simulink model "PLL_type2"  (R2014b)
settings: Solver=VariableStepDiscrete  StartTime=0.0  StopTime=50000/fs  RelTol=1e-3
PreLoadFcn:
  | %%%%%%%%%%%%%%%%%%%%%%%%%%%%%%%%%%%%%%%%%%%%%%%%%%%%%%%%%%%%%%%%%%%%%%%%%%%
  | % check to see if Simulink library folder is missing from the MATLAB path %
  | %%%%%%%%%%%%%%%%%%%%%%%%%%%%%%%%%%%%%%%%%%%%%%%%%%%%%%%%%%%%%%%%%%%%%%%%%%%
  | if isempty(strfind(path, 'rtlsdr_book_library'))
  | 
  |     % create error window
  |     fig_error = figure(...
  |         'Name', 'Error: RTL-SDR Book Library',...
  |         'Toolbar','none',...
  |         'MenuBar','none',...
  |         'NumberTitle','off',...
  |         'Resize','off',...
  |         'WindowStyle','modal');
  |     fig_error.Position(3) = 600;
  |     fig_error.Position(4) = 150;
  |     fig_axes = axes(...
  |         'Parent',fig_error,...
  |         'Position',[0,0,1,1],...
  |         'visible','off');
  |     % error message
  |     t_title = text(.05,.8,...
  |         'MISSING DIRECTORIES',...
  |         'FontSize',11.5);
  |     t_body = text(.075,.6,...
  |         [{'Simulink cannot find the  \it{<root>}\rm / \it{rtlsdr\_book\_library}\rm  folder in the \it{MATLAB Path}\rm.'},...
  |         {'Please set the MATLAB path following the instructions given in Exercise 2.4.'}],...
  |         'FontSize',10.5);
  |     % buttons
  |     btn_path = uicontrol(...
  |         'Parent',fig_error,...
  |         'String','Set Path Now',...
  |         'FontSize',10,...
  |         'Callback', 'pathtool; close(fig_error);',...
  |         'Position', [fig_error.Position(3)/2-210, 30, 200, 30]);
  |     btn_abort = uicontrol(...
  |         'Parent',fig_error,...
  |         'String','No thanks',...
  |         'FontSize',10,...
  |         'Callback', 'close(fig_error); abort=1;',...
  |         'Position', [fig_error.Position(3)/2+10, 30, 200, 30]);
  | 
  |     % pause to allow user to interact with error box
  |     uiwait(fig_error);
  | 
  |     % abort simulation
  |     try
  |         if abort==1
  |             set_param(gcs, 'SimulationCommand', 'stop');
  |         end
  |     end
  | 
  |     % if user has set path, allow diagram to be updated
  |     if ~exist('abort','var')
  |         % create error window
  |         fig_update = figure(...
  |             'Name', 'Update Diagram',...
  |             'Toolbar','none',...
  |             'MenuBar','none',...
  |             'NumberTitle','off',...
  |             'Resize','off');
  |         fig_update.Position(3) = 400;
  |         fig_update.Position(4) = 120;
  |         fig_axes = axes(...
  |             'Parent',fig_update,...
  |             'Position',[0,0,1,1],...
  |             'visible','off');
  |         % instruction message
  |         t_body = text(.075,.7,...
  |             'Once you have set the path, update the block diagram',...
  |             'FontSize',10.5);
  |         % button
  |         btn_update = uicontrol(...
  |             'Parent',fig_update,...
  |             'String','Update Block Diagram',...
  |             'FontSize',10,...
  |             'Callback', 'set_param(gcs,''SimulationCommand'',''update''); close(gcf)',...
  |             'Position', [fig_update.Position(3)/2-100, 30, 200, 30]);
  |     end
  | 
  |     % clear error components
  |     clear('fig_error','fig_update','fig_axes','t_title','t_body','btn_path','btn_abort','btn_update','abort');
  | 
  | end
  | %%%%%%%%%%%%%%%%%%%%%%%%%%%%%%%%%%%%%%%%%%%%%%%%%%%%%%%%%%%%%%%%%%%%%%%%%%%
  | 
  | 
  | MHz = 100;
  | fs = MHz * 1e6;
StartFcn:
  | close all;
StopFcn:
  | doFFTplot(fs, [Synthesised(round(length(Synthesised)*0.9):end), Error(round(length(Error)*0.9):end), Reference(round(length(Reference)*0.9):end)], ['Synthesised'; 'Error      '; 'Reference  '], 1, 7, 'hann');
  | set(7,'Name','FFT Plots of Input and Synthesised Sine Waves (Final 10% of Simulation Time)','NumberTitle','off');
  | setStandardFigSize(7);
  | legend('Error','Synthesised','Reference','location','NorthEast');
  | 
  | figure(8)
  | plot(1e6*Inst_freq.time,1e-6*Inst_freq.signals.values,'m');
  | xlabel('Time (\mus)');
  | ylabel('Frequency (MHz)');
  | title('PLL Adapting');
  | grid on;
  | 
  | set(8,'Name','Frequency Generated by VCO','NumberTitle','off');
  | setStandardFigSize(8);
undefined symbols (not defined in the file): startfcn_time_scope
libraries: commsynccomp2 x2, simulink x1, rtlsdr_book_library x1
CloseFcn:
  | closefcn_model;
Description:
  | Software, Simulation Examples and Design Exercises Licence Agreement
  | 
  | This license agreement refers to the simulation examples, design exercises and files,
  | and associated software MATLAB and Simulink resources that accompany the book:
  | 
  |      Title: Software Defined Radio using MATLAB & Simulink and the RTL-SDR
  |      Published by Strathclyde Academic Media, 2015
  |      Authored by Robert W. Stewart, Kenneth W. Barlee, Dale S.W. Atkinson,
  |      and Louise H. Crockett
  | 
  | and made available as a download from, www.desktopSDR.com or variously acquired
  | by other means such as via USB storage, cloud storage, disk or any other electronic
  | or optical or magnetic storage mechanism. These files and associated software may
  | be used subject to the terms of agreement of the conditions below:
  | 
  |     Copyright © 2015 Robert W. Stewart, Kenneth W. Barlee, Dale S.W. Atkinson,
  |     and Louise H. Crockett
  |     All rights reserved.
  | 
  | Redistribution and use in source and binary forms, with or without modification, are
  | permitted provided that the following conditions are met:
  | 
  |    1.  Redistributions of source code must retain the above copyright notice, this list of
  |         conditions and the following disclaimer.
  | 
  |    2.  Redistributions in binary form must reproduce the above copyright notice, this
  |         list of conditions and the following disclaimer in the documentation and/or other
  |         materials provided with the distribution.
  | 
  |    3.  Neither the name of the copyright holder nor the names of its contributors may
  |         be used to endorse or promote products derived from this software without
  |         specific prior written permission.
  | 
  |    4.  In all cases, the software is, and all modifications and derivatives of the
  |         software shall be, licensed to you solely for use in conjunction with The
  |         MathWorks, Inc. products and service offerings.
  | 
  | THIS SOFTWARE IS PROVIDED BY THE COPYRIGHT HOLDERS AND CONTRIBUTORS
  | "AS IS" AND ANY EXPRESS OR IMPLIED WARRANTIES, INCLUDING, BUT NOT LIMITED
  | TO, THE IMPLIED WARRANTIES OF MERCHANTABILITY AND FITNESS FOR A
  | PARTICULAR PURPOSE ARE DISCLAIMED. IN NO EVENT SHALL THE COPYRIGHT
  | HOLDER OR CONTRIBUTORS BE LIABLE FOR ANY DIRECT, INDIRECT, INCIDENTAL,
  | SPECIAL, EXEMPLARY, OR CONSEQUENTIAL DAMAGES (INCLUDING, BUT NOT
  | LIMITED TO, PROCUREMENT OF SUBSTITUTE GOODS OR SERVICES; LOSS OF USE,
  | DATA, OR PROFITS; OR BUSINESS INTERRUPTION) HOWEVER CAUSED AND ON ANY
  | THEORY OF LIABILITY, WHETHER IN CONTRACT, STRICT LIABILITY, OR TORT
  | (INCLUDING NEGLIGENCE OR OTHERWISE) ARISING IN ANY WAY OUT OF THE USE
  | OF THIS SOFTWARE, EVEN IF ADVISED OF THE POSSIBILITY OF SUCH DAMAGE.
  | 
  | 
  | Audio Tracks used in Simulations Examples and Design Exercises
  | 
  | The music and vocal files used within the Examples files and software within the book
  | were variously written, arranged, performed, recorded and produced by Garrey Rice,
  | Adam Struth, Jamie Struth, Iain Thistlethwaite and also Marshall Craigmyle who
  | collectively, and individually where appropriate, assert and retain all of their copyright,
  | performance and artistic rights. Permission to use and reproduce this music is
  | granted for all purposes associated with MATLAB and Simulink software and the
  | simulation examples and design exercises files that accompany this book. Requests to
  | use the music for any other purpose should be directed to: info@desktopSDR.com.
  | For information on music track names, full credits, and links to the musicians please
  | refer to www.desktopSDR.com/more/audio.
settings Model: Creator=desktopSDR Team  LastModifiedBy=desktopSDR Team
settings DataIOCC: LimitDataPoints=off  SaveOutput=off  SignalLogging=off  SaveTime=off
settings DebuggingCC: UnderspecifiedInitializationDetection=Classic  MergeDetectMultiDrivingBlocksExec=none

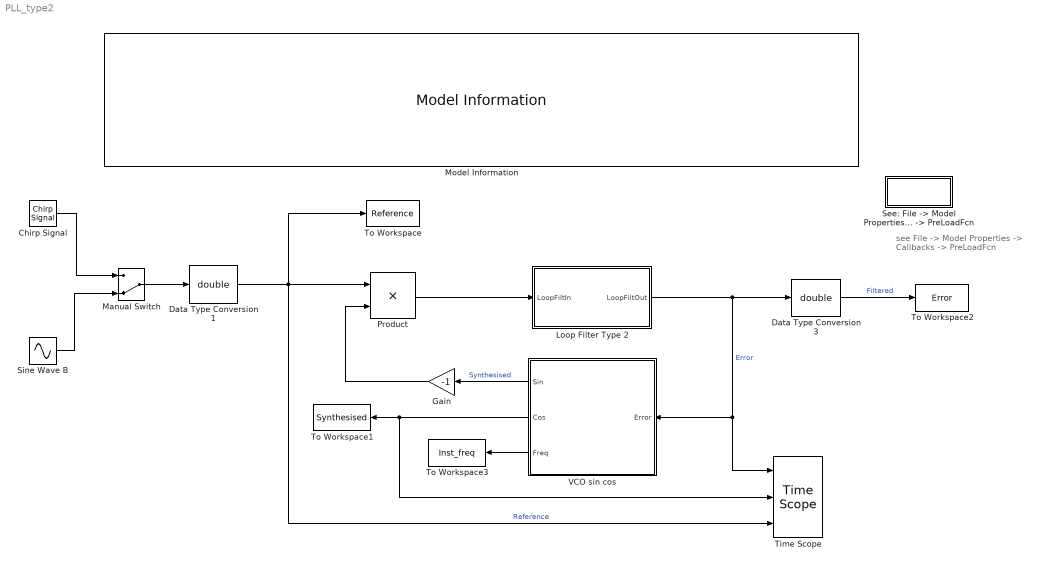
== system PLL_type2 ==
  note: see File -> Model Properties
      | -> Callbacks -> PreLoadFcn
  Chirp Signal : simulink/Sources/Chirp Signal  f1=3.6e6  T=100e3/fs  f2=3.8e6
  Data Type Conversion1 : DataTypeConversion  OutDataTypeStr=double  SampleTime=1/fs
  Data Type Conversion3 : DataTypeConversion  OutDataTypeStr=double  SampleTime=1/fs
  Gain : Gain  Gain=-1
  Loop Filter Type 2 : Subsystem  mask(Loop Filter (Type 2)){K1=0.03125, K2=1.25e-4}
      mask prompts: K1 "K1 (proportional path)"; K2 "K2 (integral path)"
      mask help: This loop filter contains two paths: a proportional path with scaling coefficient K1, and an integral path with scaling coefficient K2.
  Manual Switch : ManualSwitch  CurrentSetting=0
  Model Information : rtlsdr_book_library/Additional Tools/Model Information/Model Information
  Product : Product
  "See: File -> Model Properties -> Callbacks -> PreLoadFcn " : Subsystem
      mask Display:
      | MHz = evalin('base', 'MHz');
      | fprintf(['fs = ',num2str(MHz),' MHz']);
  Sine Wave B : Sin  Frequency=2*pi*3.55e6  Phase=pi/5  SampleTime=0
  Time Scope : TimeScope  StartFcn=startfcn_time_scope;  DefaultConfigurationName=spbscopes.TimeScopeBlockCfg  NumInputPorts=3
  To Workspace : ToWorkspace  VariableName=Reference  SampleTime=-1
  To Workspace1 : ToWorkspace  VariableName=Synthesised  SampleTime=-1
  To Workspace2 : ToWorkspace  VariableName=Error  SampleTime=-1
  To Workspace3 : ToWorkspace  VariableName=Inst_freq  SaveFormat=Structure With Time  SampleTime=-1
  VCO sin cos : Subsystem  mask(Quadratude VCO){fq=3.5e6, sensitivity=1e6}
      mask prompts: fq "Quiescent Frequency (Hz)"; sensitivity "Sensitivity (Hz/V)"
      mask help: This VCO provides both cosine and sine outputs. The quiescent frequency and sensitivity of the VCO can be defined via the mask (and these apply to both sine and cosine outputs). The block also provides the instantaneous frequency as an output.
  wires:
  Data Type Conversion1/1 -> Time Scope/3, Product/1, To Workspace/1  "Reference"
  Data Type Conversion3/1 -> To Workspace2/1  "Filtered"
  Loop Filter Type 2/1(LoopFiltOut) -> VCO sin cos/1(Error), Time Scope/1, Data Type Conversion3/1  "Error"
  Sine Wave B/1 -> Manual Switch/2
  Manual Switch/1 -> Data Type Conversion1/1
  Chirp Signal/1 -> Manual Switch/1
  Product/1 -> Loop Filter Type 2/1(LoopFiltIn)
  VCO sin cos/3(Freq) -> To Workspace3/1
  VCO sin cos/2(Cos) -> Time Scope/2, To Workspace1/1
  VCO sin cos/1(Sin) -> Gain/1  "Synthesised"
  Gain/1 -> Product/2

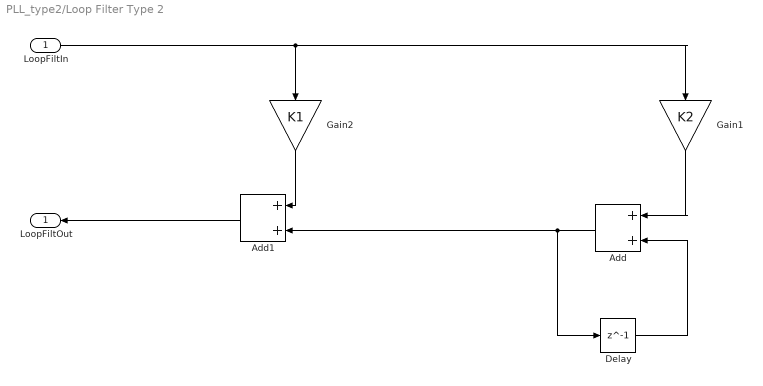
== system PLL_type2/Loop Filter Type 2 ==
  LoopFiltIn : Inport
  Add : Sum
  Add1 : Sum
  Delay : Delay  DelayLength=1
  Gain1 : Gain  Gain=K2
  Gain2 : Gain  Gain=K1
  LoopFiltOut : Outport
  wires:
  Add1/1 -> LoopFiltOut/1
  Delay/1 -> Add/2
  Add/1 -> Delay/1, Add1/2
  LoopFiltIn/1 -> Gain2/1, Gain1/1
  Gain2/1 -> Add1/1
  Gain1/1 -> Add/1

== system PLL_type2/See: File -> Model Properties -> Callbacks -> PreLoadFcn  ==

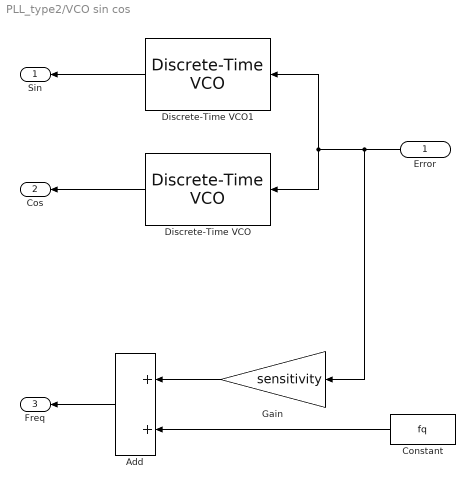
== system PLL_type2/VCO sin cos ==
  Error : Inport
  Add : Sum
  Constant : Constant  Value=fq
  Discrete-Time VCO : commsynccomp2/Discrete-Time VCO  Ac=1  Fc=fq  Kc=sensitivity  Ph=pi/2  ts=1/fs
  Discrete-Time VCO1 : commsynccomp2/Discrete-Time VCO  Ac=1  Fc=fq  Kc=sensitivity  Ph=0  ts=1/fs
  Gain : Gain  Gain=sensitivity
  Sin : Outport
  Cos : Outport  Port=2
  Freq : Outport  Port=3
  wires:
  Discrete-Time VCO1/1 -> Sin/1
  Discrete-Time VCO/1 -> Cos/1
  Error/1 -> Gain/1, Discrete-Time VCO/1, Discrete-Time VCO1/1
  Gain/1 -> Add/1
  Constant/1 -> Add/2
  Add/1 -> Freq/1
